simulink model "AOE_OBAS"  (R2024b)
settings: Solver=ode4  StartTime=0  StopTime=200  FixedStep=0.01  MaxStep=0.01  RelTol=1e-3
values from neighbouring files (symbols this model uses):
  AOE = Constants_3Body_v2(inputs)    [wecSimInputFile.m]
undefined symbols (not defined in the file or in its folder): body, constraint, DiscIntNeverNeededParam, pto
libraries: WECSim_Lib_Body_Elements x6, simulink x3, WECSim_Lib_Constraints x3, WECSim_Lib_PTOs x3, WECSim_Lib_Frames x1
(part 1 of 2)
settings Model: Creator=wcwi  LastModifiedBy=Luke
settings SolverCC: ZeroCrossControl=DisableAll  AlgebraicLoopSolver=TrustRegion  PositivePriorityOrder=on  AutoInsertRateTranBlk=on  InsertRTBMode=Never (minimum delay)
settings DataIOCC: SaveFormat=Array  ReturnWorkspaceOutputs=off
settings OptimizationCC: LifeSpan=inf  SimCompilerOptimization=on  AccelVerboseBuild=on
settings DebuggingCC: UnconnectedInputMsg=warning  UnconnectedOutputMsg=warning  UnconnectedLineMsg=warning  SFUnexpectedBacktrackingDiag=warning  SFNoUnconditionalDefaultTransitionDiag=warning  SFExecutionAtInitializationDiag=none  ArithmeticOperatorsInVariantConditions=warning
settings HardwareCC: ProdBitPerSizeT=32  ProdBitPerPtrDiffT=32  ProdWordSize=32  ProdHWDeviceType=Specified
settings ModelReferenceCC: UpdateModelReferenceTargets=Force  PropagateSignalLabelsOutOfModel=off
settings SFSimCC: SimUseLocalCustomCode=off  CustomCodeUndefinedFunction=UseInterfaceOnly
settings RTWCC: RTWUseLocalCustomCode=off  GPUComputeCapability=3.5
settings CodeAppCC: StateflowObjectComments=on
settings GRTTargetCC: TargetLangStandard=C89/C90 (ANSI)
settings ConfigComp: CovMetricSettings=dw  CovSaveCumulativeToWorkspaceVar=on  CovSaveSingleToWorkspaceVar=on  CovExternalEMLEnable=off

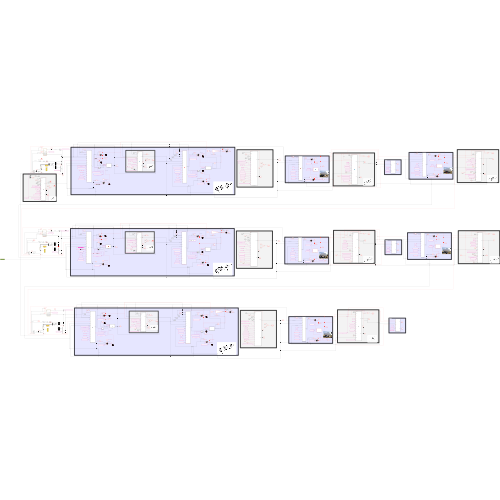
[thumbnail: Simulink's stored preview of the top-level diagram]
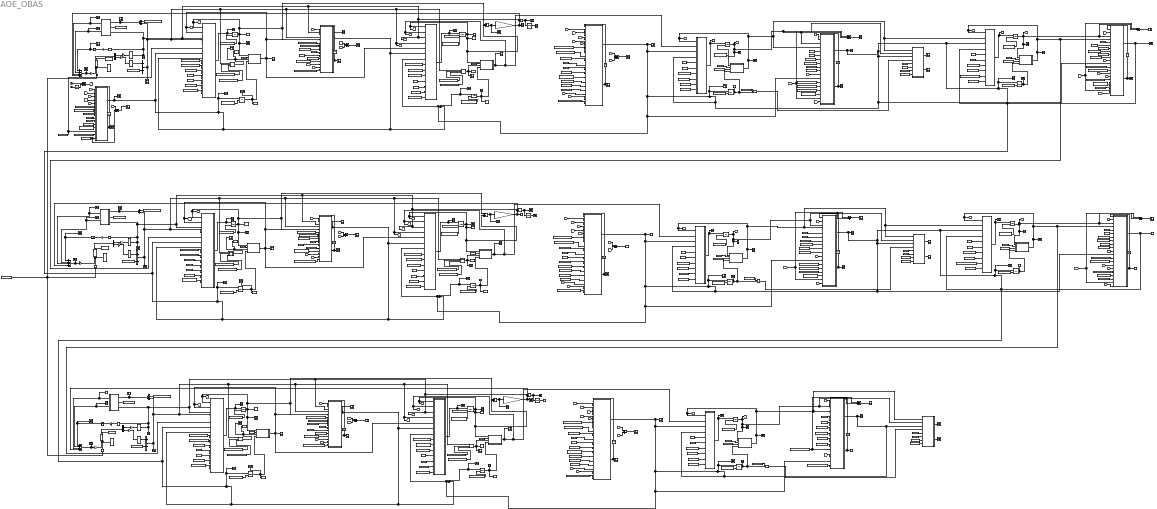
== system AOE_OBAS ==
  note: Outlet Piston Chamber 1 Valve
  note: Outlet Tank Valve
  note: Inlet Piston valve
  note: Outlet Piston Valve
  note: Outlet Piston Chamber 1 Valve
  note: Outlet Tank Valve
  note: Outlet Piston Valve
  note: Outlet Piston Chamber 1 Valve
  note: Outlet Tank Valve
  note: Outlet Piston Valve
  note: Useful Power
  note: Useful Power
  note: Useful Power
  note: Outlet Tank Valve
  note: Outlet Tank Valve
  " mdot Pipe U1U2" : Scope
  " mdot Pipe U2U3" : Scope
  " mdot Tank Unit1" : Scope
  " mdot Tank Unit2" : Scope
  " mdot Tank Unit3" : Scope
  " mdot max Pipe U1U2" : Scope
  " mdot max Pipe U2U3" : Scope
  " mdot max Tank Unit1" : Scope
  " mdot max Tank Unit2" : Scope
  " mdot max Tank Unit3" : Scope
  Add{1,13..15} (4 alike) : Sum  Inputs=+-
  Add{2..7,9..11,16..18} (12 alike) : Sum  Inputs=-+
  Add12 : Sum  Inputs=++++  RndMeth=Simplest
  Add19 : Sum  Inputs=++++  RndMeth=Simplest
  Add8 : Sum  Inputs=++++  RndMeth=Simplest
  Air Mass Chamber1 Unit1 : Scope
  Air Mass Chamber1 Unit2 : Scope
  Air Mass Chamber1 Unit3 : Scope
  Air Mass Chamber2 Unit1 : Scope
  Air Mass Chamber2 Unit2 : Scope
  Air Mass Chamber2 Unit3 : Scope
  Air Mass Pipe U1U2 : Scope
  Air Mass Pipe U2U3 : Scope
  Air Mass change rate Chamber1 Unit1 : Scope
  Air Mass change rate Chamber1 Unit2 : Scope
  Air Mass change rate Chamber1 Unit3 : Scope
  Air Mass change rate Chamber2 Unit1 : Scope
  Air Mass change rate Chamber2 Unit2 : Scope
  Air Mass change rate Chamber2 Unit3 : Scope
  Assertion : Assertion  AssertionFailFcn=Ch1C1 mass is zero
  Assertion1 : Assertion  AssertionFailFcn=Ch1C1 pressure is zero
  Assertion10 : Assertion  AssertionFailFcn=Ch1C1 volume is zero
  Assertion11 : Assertion  AssertionFailFcn=Ch2C1 volume is zero
  Assertion12 : Assertion  AssertionFailFcn=Ch1C1 mass is zero
  Assertion13 : Assertion  AssertionFailFcn=Ch1C1 pressure is zero
  Assertion14 : Assertion  AssertionFailFcn=Ch2C1 pressure is zero  StopWhenAssertionFail=off
  Assertion15 : Assertion  AssertionFailFcn=Ch2C1 mass is zero
  Assertion16 : Assertion  AssertionFailFcn=Ch1C1 volume is zero
  Assertion17 : Assertion  AssertionFailFcn=Ch2C1 volume is zero
  Assertion2 : Assertion  AssertionFailFcn=Ch2C1 pressure is zero  StopWhenAssertionFail=off
  Assertion3 : Assertion  AssertionFailFcn=Ch2C1 mass is zero
  Assertion4 : Assertion  AssertionFailFcn=Ch1C1 volume is zero
  Assertion5 : Assertion  AssertionFailFcn=Ch2C1 volume is zero
  Assertion6 : Assertion  AssertionFailFcn=Ch1C1 mass is zero
  Assertion7 : Assertion  AssertionFailFcn=Ch1C1 pressure is zero
  Assertion8 : Assertion  AssertionFailFcn=Ch2C1 pressure is zero  StopWhenAssertionFail=off
  Assertion9 : Assertion  AssertionFailFcn=Ch2C1 mass is zero
  Atmospheric pressure{1..4} (4 alike) : Constant  Value=AOE.AtmPressure
  Bus Selector : BusSelector  OutputSignals=velocity,position
  Bus Selector1 : BusSelector  OutputSignals=velocity,position
  Bus Selector2 : BusSelector  OutputSignals=velocity,position
  Chamber pressure potential Unit1 : Scope
  Chamber pressure potential Unit2 : Scope
  Chamber pressure potential Unit3 : Scope
  Clock : Clock
  Clock1 : Clock
  Constant{1,14,24,37,56} (5 alike) : Constant  Value=AOE.Unit1.Cylinder.HeatConvection
  Constant{2,10,71,85,208} (5 alike) : Constant  Value=AOE.Unit2.Cylinder.HeatConvection
  Constant{76,90,94,97,100,118,200} (7 alike) : Constant  Value=AOE.Unit2.Cylinder.CrossSectionalArea
  Constant{8,26,38,42,52,57,64,73,86,91,101,106,119,133,146,151,161,166,174,179,186,209,214} (23 alike) : Constant  Value=AOE.WaterTemperature
  Constant102 : Constant  Value=AOE.Unit2.Tank.HeatConvection
  Constant103 : Constant  Value=AOE.Unit2.Tank.SurfaceArea
  Constant{96,99,104,110} (4 alike) : Constant  Value=AOE.Unit2.Tank.Volume
  Constant105 : Constant  Value=AOE.Unit1.Pipe.CrossSectionalArea
  Constant107 : Constant  Value=AOE.Unit2.Tank.HeatConvection
  Constant108 : Constant  Value=AOE.Unit2.Tank.SurfaceArea
  Constant{6,23,28,31,40,47,62,70,75,79,89,95,109,130,135,139,149,155,169,181,198,203,213} (23 alike) : Constant  Value=AOE.gma
  Constant11 : Constant  Value=AOE.Unit2.Chamber2.InitialPistonPosition
  Constant111 : Constant  Value=AOE.Unit1.Pipe.HeatConvection
  Constant112 : Constant  Value=AOE.Unit2.Pipe.InitialAirMass
  Constant113 : Constant  Value=AOE.Unit2.Pipe.CrossSectionalArea
  Constant{3..5,22,27,30,35,39,43,61,69,74,77..78,83,87..88,92,98,114,129,134,137..138,143,147..148,152,158,165,172,175,185,197,202,207,211} (37 alike) : Constant  Value=AOE.Rs
  Constant115 : Constant  Value=AOE.Cp
  Constant116 : Constant  Value=AOE.Unit2.OutletCylinderOrifice.CrossSectionalArea
  Constant117 : Constant  Value=AOE.Unit2.Chamber1Chamber2Orifice.CrossSectionalArea
  Constant12 : Constant  Value=AOE.Unit2.Cylinder.Diameter
  Constant120 : Constant  Value=AOE.Unit2.Chamber1.InitialAirMass
  Constant{121..122,131,145,195} (5 alike) : Constant  Value=AOE.Unit3.Cylinder.HeatConvection
  Constant123 : Constant  Value=AOE.Unit3.Chamber2.InitialPistonPosition
  Constant124 : Constant  Value=AOE.Unit3.Cylinder.Diameter
  Constant125 : Constant  Value=AOE.Unit3.Chamber2.InitialAirMass
  Constant126 : Constant  Value=AOE.Unit3.Chamber1.InitialPressure
  Constant127 : Constant  Value=AOE.Unit3.Chamber2.InitialPressure
  Constant128 : Constant  Value=AOE.Unit3.OutletTankOrifice.CrossSectionalArea
  Constant13 : Constant  Value=AOE.Unit2.Chamber2.InitialAirMass
  Constant132 : Constant  Value=AOE.Unit3.Tank.InitialAirMass
  Constant{136,150,154,157,160,178,194} (7 alike) : Constant  Value=AOE.Unit3.Cylinder.CrossSectionalArea
  Constant140 : Constant  Value=AOE.Unit3.Tank.HeatConvection
  Constant141 : Constant  Value=AOE.Unit3.Tank.InitialPressure
  Constant142 : Constant  Value=AOE.Unit3.Tank.SurfaceArea
  Constant{36,48,50,55,60,84,144} (7 alike) : Constant  Value=AOE.Unit1.Tank.Volume
  Constant15 : Constant  Value=AOE.Unit2.Chamber1.InitialPressure
  Constant153 : Constant  Value=AOE.Unit3.Chamber2.InitialPistonPosition
  Constant{156,159,164,170} (4 alike) : Constant  Value=AOE.Unit3.Tank.Volume
  Constant16 : Constant  Value=AOE.Unit1.Chamber2.InitialPistonPosition
  Constant162 : Constant  Value=AOE.Unit3.Tank.HeatConvection
  Constant163 : Constant  Value=AOE.Unit3.Tank.SurfaceArea
  Constant167 : Constant  Value=AOE.Unit3.Tank.HeatConvection
  Constant168 : Constant  Value=AOE.Unit3.Tank.SurfaceArea
  Constant17 : Constant  Value=AOE.Unit1.Cylinder.Diameter
  Constant171 : Constant  Value=AOE.Cp
  Constant173 : Constant  Value=AOE.Cp
  Constant176 : Constant  Value=AOE.Unit3.OutletCylinderOrifice.CrossSectionalArea
  Constant177 : Constant  Value=AOE.Unit3.Chamber1Chamber2Orifice.CrossSectionalArea
  Constant18 : Constant  Value=AOE.Unit1.Chamber2.InitialAirMass
  Constant180 : Constant  Value=AOE.Unit3.Chamber1.InitialAirMass
  Constant182 : Constant  Value=AOE.Unit2.Pipe.HeatConvection
  Constant183 : Constant  Value=AOE.Unit2.Pipe.InitialPressure
  Constant184 : Constant  Value=AOE.Unit2.Pipe.SurfaceArea
  Constant{187..188,193,199} (4 alike) : Constant  Value=AOE.Unit2.Pipe.Volume
  Constant189 : Constant  Value=AOE.Unit2.Pipe.HeatConvection
  Constant19 : Constant  Value=AOE.Unit1.Chamber1.InitialPressure
  Constant190 : Constant  Value=AOE.Unit2.Pipe.SurfaceArea
  Constant191 : Constant  Value=AOE.Unit2.Pipe.HeatConvection
  Constant196 : Constant  Value=AOE.Unit2.OutletPipeOrifice.CrossSectionalArea
  Constant20 : Constant  Value=AOE.Unit1.Chamber2.InitialPressure
  Constant201 : Constant  Value=AOE.Unit1.Pipe.InitialAirMass
  Constant204 : Constant  Value=AOE.Unit1.Pipe.HeatConvection
  Constant205 : Constant  Value=AOE.Unit1.Pipe.InitialPressure
  Constant206 : Constant  Value=AOE.Unit1.Pipe.SurfaceArea
  Constant21 : Constant  Value=AOE.Unit1.OutletTankOrifice.CrossSectionalArea
  Constant210 : Constant  Value=AOE.Unit1.OutletPipeOrifice.CrossSectionalArea
  Constant{212,217..218,220} (4 alike) : Constant  Value=AOE.Unit1.Pipe.Volume
  Constant215 : Constant  Value=AOE.Unit1.Pipe.HeatConvection
  Constant216 : Constant  Value=AOE.Unit1.Pipe.SurfaceArea
  Constant25 : Constant  Value=AOE.Unit1.Tank.InitialAirMass
  Constant{7,29,41,46,49,51,63} (7 alike) : Constant  Value=AOE.Unit1.Cylinder.CrossSectionalArea
  Constant32 : Constant  Value=AOE.Unit1.Tank.HeatConvection
  Constant33 : Constant  Value=AOE.Unit1.Tank.InitialPressure
  Constant34 : Constant  Value=AOE.Unit1.Tank.SurfaceArea
  Constant44 : Constant  Value=AOE.Unit1.Chamber2.InitialPistonPosition
  Constant45 : Constant  Value=AOE.Unit2.Chamber2.InitialPressure
  Constant53 : Constant  Value=AOE.Unit1.Tank.HeatConvection
  Constant54 : Constant  Value=AOE.Unit1.Tank.SurfaceArea
  Constant58 : Constant  Value=AOE.Unit1.Tank.HeatConvection
  Constant59 : Constant  Value=AOE.Unit1.Tank.SurfaceArea
  Constant65 : Constant  Value=AOE.Unit1.InletCylinderOrifice.CrossSectionalArea
  Constant66 : Constant  Value=AOE.Unit1.OutletCylinderOrifice.CrossSectionalArea
  Constant67 : Constant  Value=AOE.Unit1.Chamber1Chamber2Orifice.CrossSectionalArea
  Constant68 : Constant  Value=AOE.Unit2.OutletTankOrifice.CrossSectionalArea
  Constant72 : Constant  Value=AOE.Unit2.Tank.InitialAirMass
  Constant80 : Constant  Value=AOE.Unit2.Tank.HeatConvection
  Constant81 : Constant  Value=AOE.Unit2.Tank.InitialPressure
  Constant82 : Constant  Value=AOE.Unit2.Tank.SurfaceArea
  Constant9 : Constant  Value=AOE.Unit1.Chamber1.InitialAirMass
  Constant93 : Constant  Value=AOE.Unit2.Chamber2.InitialPistonPosition
  Coulomb & Viscous Friction Unit1 : simulink/Discontinuities/Coulomb & Viscous Friction  offset=0  gain=AOE.Unit1.Cylinder.CoulombFrictionGain
  Coulomb & Viscous Friction Unit2 : simulink/Discontinuities/Coulomb & Viscous Friction  offset=0  gain=AOE.Unit1.Cylinder.CoulombFrictionGain
  Coulomb & Viscous Friction Unit3 : simulink/Discontinuities/Coulomb & Viscous Friction  offset=0  gain=AOE.Unit1.Cylinder.CoulombFrictionGain
  Cyl D{,1..3} (4 alike) : Constant  Value=AOE.Unit1.Cylinder.Diameter
  Cyl D{6,8..9,11} (4 alike) : Constant  Value=AOE.Unit3.Cylinder.Diameter
  Cyl D{4..5,7,13} (4 alike) : Constant  Value=AOE.Unit2.Cylinder.Diameter
  Determining Useful Energy : MATLAB Function
      settings: MinAlgLoopOccurrences=on
  Determining Useful Energy1 : MATLAB Function
      settings: MinAlgLoopOccurrences=on
  Determining Useful Energy2 : MATLAB Function
      settings: MinAlgLoopOccurrences=on
  Discrete-Time Integrator{,1,3,5,8,12..15,18,21} (11 alike) : DiscreteIntegrator  InitialConditionSource=external  InitialCondition=101.3  SampleTime=-1  LimitOutput=on  LowerSaturationLimit=0  ICPrevOutput=DiscIntNeverNeededParam  ICPrevScaledInput=DiscIntNeverNeededParam
  Discrete-Time Integrator{4,6,10,16,20} (5 alike) : DiscreteIntegrator  InitialConditionSource=external  InitialCondition=1.2754*(10)*.25*pi*0.5^2  SampleTime=-1  LimitOutput=on  LowerSaturationLimit=0  ICPrevOutput=DiscIntNeverNeededParam  ICPrevScaledInput=DiscIntNeverNeededParam
  Discrete-Time Integrator{2,7,9,11,17,19} (6 alike) : DiscreteIntegrator  InitialConditionSource=external  InitialCondition=1.2754*(2+.05)*.25*pi*2.14^2  SampleTime=-1  LimitOutput=on  LowerSaturationLimit=0  ICPrevOutput=DiscIntNeverNeededParam  ICPrevScaledInput=DiscIntNeverNeededParam
  Endstop Forces Unit1 : Subsystem
  Endstop Forces Unit2 : Subsystem
  Endstop Forces Unit3 : Subsystem
  Energy : DiscreteIntegrator  SampleTime=-1  LimitOutput=on  ICPrevOutput=DiscIntNeverNeededParam  ICPrevScaledInput=DiscIntNeverNeededParam
  Energy Unit1 : Scope
  Energy Unit2 : Scope
  Energy Unit3 : Scope
  Energy1 : DiscreteIntegrator  SampleTime=-1  LimitOutput=on  ICPrevOutput=DiscIntNeverNeededParam  ICPrevScaledInput=DiscIntNeverNeededParam
  Energy2 : DiscreteIntegrator  SampleTime=-1  LimitOutput=on  ICPrevOutput=DiscIntNeverNeededParam  ICPrevScaledInput=DiscIntNeverNeededParam
  Exergy Unit1 : Scope
  Exergy Unit2 : Scope
  Exergy Unit3 : Scope
  Float : WECSim_Lib_Body_Elements/Rigid Body  body=body(1)
  Float1 : WECSim_Lib_Body_Elements/Rigid Body  body=body(3)
  Float2 : WECSim_Lib_Body_Elements/Rigid Body  body=body(5)
  Floating (6DOF) : WECSim_Lib_Constraints/Floating (6DOF)  constraint=constraint(1)
      settings: AttributesFormatString=%<constraint>
  Floating (6DOF)1 : WECSim_Lib_Constraints/Floating (6DOF)  constraint=constraint(2)
      settings: AttributesFormatString=%<constraint>
  Floating (6DOF)2 : WECSim_Lib_Constraints/Floating (6DOF)  constraint=constraint(3)
      settings: AttributesFormatString=%<constraint>
  Gain{,2,4,6..14} (12 alike) : Gain  Gain=-1
  Gain1 : Gain  Gain=AOE.Unit1.Cylinder.CrossSectionalArea
  Gain3 : Gain  Gain=AOE.Unit2.Cylinder.CrossSectionalArea
  Gain5 : Gain  Gain=AOE.Unit3.Cylinder.CrossSectionalArea
  Global Reference Frame : WECSim_Lib_Frames/Global Reference Frame  waves=waves  simu=simu
      settings: SourceProductName=WEC-Sim
  Mech_Energy Unit1 : Scope
  Mech_Energy Unit2 : Scope
  Mech_Energy Unit3 : Scope
  Mech_FTO Unit1 : Scope
  Mech_FTO Unit2 : Scope
  Mech_FTO Unit3 : Scope
  Mech_PTO Unit1 : Scope
  Mech_PTO Unit2 : Scope
  Mech_PTO Unit3 : Scope
  PTO Friction Unit1 : Scope
  PTO Friction Unit2 : Scope
  PTO Friction Unit3 : Scope
  Pdot Chamber1 Unit1 : Scope
  Pdot Chamber1 Unit2 : Scope
  Pdot Chamber1 Unit3 : Scope
  Pdot Chamber2 Unit1 : Scope
  Pdot Chamber2 Unit2 : Scope
  Pdot Chamber2 Unit3 : Scope
  Pdot Pipe U1U2 : Scope
  Pdot Pipe U2U3 : Scope
  Pdot Tank Unit1 : Scope
  Pdot Tank Unit2 : Scope
  Pdot Tank Unit3 : Scope
  Pipe Air Mass change rate U1U2 : Scope
  Pipe Air Mass change rate U2U3 : Scope
  Pipe Unit1 to Unit1 : MATLAB Function
      settings: MinAlgLoopOccurrences=on
  Pipe Unit1 to Unit2 : MATLAB Function
      settings: MinAlgLoopOccurrences=on
  Pressure Chamber1 Box Unit1 : MATLAB Function
      settings: MinAlgLoopOccurrences=on
  Pressure Chamber1 Box Unit2 : MATLAB Function
      settings: MinAlgLoopOccurrences=on
  Pressure Chamber1 Box Unit3 : MATLAB Function
      settings: MinAlgLoopOccurrences=on
  Pressure Chamber1 Unit1 : Scope
  Pressure Chamber1 Unit2 : Scope
  Pressure Chamber1 Unit3 : Scope
  Pressure Chamber2 Box Unit1 : MATLAB Function
  Pressure Chamber2 Box Unit2 : MATLAB Function
  Pressure Chamber2 Box Unit3 : MATLAB Function
  Pressure Chamber2 Unit1 : Scope
  Pressure Chamber2 Unit2 : Scope
  Pressure Chamber2 Unit3 : Scope
  Pressure Difference Chamb. 1 Unit1 : Scope
  Pressure Difference Chamb. 1 Unit2 : Scope
  Pressure Difference Chamb. 1 Unit3 : Scope
  Pressure Difference Cyl. Unit1 : Scope
  Pressure Difference Cyl. Unit2 : Scope
  Pressure Difference Cyl. Unit3 : Scope
  Pressure Difference Inlet Unit1 : Scope
  Pressure Difference Pipe U2U3 : Scope
  Pressure Difference Pipe Unit1 : Scope
  Pressure Difference Tank Unit1 : Scope
  Pressure Difference Tank Unit2 : Scope
  Pressure Difference Tank Unit3 : Scope
  Pressure Pipe U1U2 : Scope
  Pressure Pipe U2U3 : Scope
  Pressure Tank Box Unit1 : MATLAB Function
      settings: MinAlgLoopOccurrences=on
  Pressure Tank Box Unit2 : MATLAB Function
      settings: MinAlgLoopOccurrences=on
  Pressure Tank Box Unit3 : MATLAB Function
      settings: MinAlgLoopOccurrences=on
  Pressure Tank Unit1 : Scope
  Pressure Tank Unit2 : Scope
  Pressure Tank Unit3 : Scope
  Product1 : Product  Inputs=/*
  Product2 : Product
  Product3 : Product  Inputs=/*
  Product4 : Product  Inputs=/*
  Product5 : Product
  Product8 : Product
  Revised Valve Model : MATLAB Function
      settings: MinAlgLoopOccurrences=on
  Revised Valve Model Chamber1Chamber2 Unit1 : MATLAB Function
      settings: MinAlgLoopOccurrences=on
  Revised Valve Model Chamber1Chamber2 Unit2 : MATLAB Function
      settings: MinAlgLoopOccurrences=on
  Revised Valve Model Chamber1Chamber2 Unit3 : MATLAB Function
      settings: MinAlgLoopOccurrences=on
  Revised Valve Model Inlet Unit1 : MATLAB Function
      settings: MinAlgLoopOccurrences=on
  Revised Valve Model Piston Outlet Unit2 : MATLAB Function
      settings: MinAlgLoopOccurrences=on
  Revised Valve Model Piston Outlet Unit3 : MATLAB Function
      settings: MinAlgLoopOccurrences=on
  Revised Valve Pipe Outlet Unit1 : MATLAB Function
      settings: MinAlgLoopOccurrences=on
  Revised Valve Pipe Outlet Unit2 : MATLAB Function
      settings: MinAlgLoopOccurrences=on
  Revised Valve Tank Outlet Unit1 : MATLAB Function
      settings: MinAlgLoopOccurrences=on
  Revised Valve Tank Outlet Unit2 : MATLAB Function
      settings: MinAlgLoopOccurrences=on
  Revised Valve Tank Outlet2 : MATLAB Function
      settings: MinAlgLoopOccurrences=on
  Saturation : Saturate  UpperLimit=AOE.Unit1.Cylinder.CoulombFrictionLimit  LowerLimit=-AOE.Unit1.Cylinder.CoulombFrictionLimit
  Saturation1 : Saturate  UpperLimit=AOE.Unit1.Cylinder.CoulombFrictionLimit  LowerLimit=-AOE.Unit1.Cylinder.CoulombFrictionLimit
  Saturation2 : Saturate  UpperLimit=AOE.Unit1.Cylinder.CoulombFrictionLimit  LowerLimit=-AOE.Unit1.Cylinder.CoulombFrictionLimit
  Selector{,1..5} (6 alike) : Selector  InputPortWidth=6  IndexOptions=Index vector (dialog)  Indices=3  OutputSizes=1
  Spar : WECSim_Lib_Body_Elements/Rigid Body  body=body(2)
  Spar1 : WECSim_Lib_Body_Elements/Rigid Body  body=body(4)
  Spar2 : WECSim_Lib_Body_Elements/Rigid Body  body=body(6)
  Sum : Sum  Inputs=+-
  Sum{1..2,5,7,11..12} (6 alike) : Sum  Inputs=-+
  Sum10 : Sum  Inputs=+-
  Sum{3,8,13,15..16} (5 alike) : Sum  Inputs=+|-
  Sum14 : Sum
  Sum4 : Sum  Inputs=+-
  Sum6 : Sum
  Sum9 : Sum
  Tank Air Mass Unit1 : Scope
  Tank Air Mass Unit2 : Scope
  Tank Air Mass Unit3 : Scope
  Tank Air Mass change rate Unit1 : Scope
  Tank Air Mass change rate Unit2 : Scope
  Tank Air Mass change rate Unit3 : Scope
  Temp Chamber1 Unit1 : Scope
  Temp Chamber1 Unit2 : Scope
  Temp Chamber1 Unit3 : Scope
  Temp Chamber2 Unit1 : Scope
  Temp Chamber2 Unit2 : Scope
  Temp Chamber2 Unit3 : Scope
  Temp Pipe U1U2 : Scope
  Temp Pipe U2U3 : Scope
  Temp Tank Unit1 : Scope
  Temp Tank Unit2 : Scope
  Temp Tank Unit3 : Scope
  Temperature Chamber1 Box Unit1 : MATLAB Function  TreatAsAtomicUnit=on
      settings: MinAlgLoopOccurrences=on
  Temperature Chamber1 Box Unit2 : MATLAB Function  TreatAsAtomicUnit=on
      settings: MinAlgLoopOccurrences=on
  Temperature Chamber1 Box Unit3 : MATLAB Function  TreatAsAtomicUnit=on
      settings: MinAlgLoopOccurrences=on
  Temperature Chamber2 Box Unit1 : MATLAB Function
      settings: MinAlgLoopOccurrences=on
  Temperature Chamber2 Box Unit2 : MATLAB Function
      settings: MinAlgLoopOccurrences=on
  Temperature Chamber2 Box Unit3 : MATLAB Function
      settings: MinAlgLoopOccurrences=on
  Temperature Pipe Unit1 to Unit1 : MATLAB Function
  Temperature Pipe Unit1 to Unit2 : MATLAB Function
  Temperature Tank Box Unit1 : MATLAB Function
  Temperature Tank Box Unit2 : MATLAB Function
  Temperature Tank Box Unit3 : MATLAB Function
  Total Reaction Force : Scope
  Total Reaction Force1 : Scope
  Total Reaction Force2 : Scope
  Translational PTO Actuation Force : WECSim_Lib_PTOs/Translational PTO Actuation Force  pto=pto(1)
      settings: AttributesFormatString=%<pto>
  Translational PTO Actuation Force1 : WECSim_Lib_PTOs/Translational PTO Actuation Force  pto=pto(2)
      settings: AttributesFormatString=%<pto>
  Translational PTO Actuation Force2 : WECSim_Lib_PTOs/Translational PTO Actuation Force  pto=pto(3)
      settings: AttributesFormatString=%<pto>
  Unit Delay{,1..12} (13 alike) : UnitDelay  SampleTime=-1  HasFrameUpgradeWarning=on
  Vol Chamber1 Unit1 : Scope
  Vol Chamber1 Unit2 : Scope
  Vol Chamber1 Unit3 : Scope
  Vol Chamber2 Unit1 : Scope
  Vol Chamber2 Unit2 : Scope
  Vol Chamber2 Unit3 : Scope
  Volume Chamber1 Box Unit1 : MATLAB Function  TreatAsAtomicUnit=on
      settings: MinAlgLoopOccurrences=on
  Volume Chamber1 Box Unit2 : MATLAB Function  TreatAsAtomicUnit=on
      settings: MinAlgLoopOccurrences=on
  Volume Chamber1 Box Unit3 : MATLAB Function  TreatAsAtomicUnit=on
      settings: MinAlgLoopOccurrences=on
  Volume Chamber2 Box Unit1 : MATLAB Function  TreatAsAtomicUnit=on
      settings: MinAlgLoopOccurrences=on
  Volume Chamber2 Box Unit2 : MATLAB Function  TreatAsAtomicUnit=on
      settings: MinAlgLoopOccurrences=on
  Volume Chamber2 Box Unit3 : MATLAB Function  TreatAsAtomicUnit=on
      settings: MinAlgLoopOccurrences=on
  cylinder equilibrium offset position{1,3..5} (4 alike) : Constant  Value=AOE.Unit1.Chamber1.InitialPistonPosition
  cylinder equilibrium offset position{7,9..10,20} (4 alike) : Constant  Value=AOE.Unit2.Chamber1.InitialPistonPosition
  cylinder equilibrium offset position{11,13,15..16} (4 alike) : Constant  Value=AOE.Unit3.Chamber1.InitialPistonPosition
  cylinder equilibrium offset position12 : Constant  Value=AOE.Unit2.Chamber2.InitialPistonPosition
  cylinder equilibrium offset position14 : Constant  Value=AOE.Unit3.Chamber2.InitialPistonPosition
  cylinder equilibrium offset position18 : Constant  Value=AOE.Unit3.Chamber2.InitialPistonPosition
  cylinder equilibrium offset position2 : Constant  Value=AOE.Unit1.Chamber2.InitialPistonPosition
  cylinder equilibrium offset position6 : Constant  Value=AOE.Unit1.Chamber2.InitialPistonPosition
  cylinder equilibrium offset position8 : Constant  Value=AOE.Unit2.Chamber2.InitialPistonPosition
  cylinder total Length : Constant  Value=AOE.Unit1.Cylinder.Length
  cylinder total Length1 : Constant  Value=AOE.Unit2.Cylinder.Length
  cylinder total Length2 : Constant  Value=AOE.Unit3.Cylinder.Length
  cylinder total Length3 : Constant  Value=AOE.Unit1.Cylinder.InitialOffset
  cylinder total Length4 : Constant  Value=AOE.Unit1.Cylinder.InitialOffset
  cylinder total Length5 : Constant  Value=AOE.Unit1.Cylinder.InitialOffset
  joint F stop high Unit1 : Scope
  joint F stop high Unit2 : Scope
  joint F stop high Unit3 : Scope
  joint F stop low Unit1 : Scope
  joint F stop low Unit2 : Scope
  joint F stop low Unit3 : Scope
  joint position1 : Scope
  joint position2 : Scope
  joint position3 : Scope
  mdot Chamber1Chamber2 Unit1 : Scope
  mdot Chamber1Chamber2 Unit2 : Scope
  mdot Chamber1Chamber2 Unit3 : Scope
  mdot Cylinder Unit1 : Scope
  mdot Cylinder Unit2 : Scope
  mdot Cylinder Unit3 : Scope
  mdot Inlet Unit1 : Scope
  mdot Max Chamber1Chamber2 Unit1 : Scope
  mdot Max Chamber1Chamber2 Unit2 : Scope
  mdot Max Chamber1Chamber2 Unit3 : Scope
  mdot Max Cylinder Unit1 : Scope
  mdot Max Cylinder Unit2 : Scope
  mdot Max Cylinder Unit3 : Scope
  mdot max Inlet Unit1 : Scope
  override3 : Constant  Value=AOE.Unit3.OutletTankCheckValve.CrackPressure
  piston position Unit1 : Scope
  piston position Unit2 : Scope
  piston position Unit3 : Scope
  piston velocity Unit2 : Scope
  piston velocity Unit3 : Scope
  piston velocity Unit4 : Scope
  tempAmb{1..4} (4 alike) : Constant  Value=AOE.AtmTemperature
  wires:
  Coulomb & Viscous Friction Unit1/1 -> Gain/1
  Saturation/1 -> PTO Friction Unit1/1, Add8/1  "Motion Friction"
  Endstop Forces Unit1/2(F_stop_lo) -> joint F stop low Unit1/1, Add8/2  "Fstop_low"
  cylinder total Length/1 -> Endstop Forces Unit1/2(Total length)
  Sum6/1 -> Endstop Forces Unit1/1(x(t)), joint position1/1  "Piston Position"
  Endstop Forces Unit1/1(F_stop_hi) -> joint F stop high Unit1/1, Add8/3  "Fstop_high"
  Gain/1 -> Saturation/1
  Constant44/1 -> Sum6/1
  Add13/1 -> piston position Unit1/1, Volume Chamber1 Box Unit1/1(x), Revised Valve Model Chamber1Chamber2 Unit1/4(x), Pressure Chamber2 Box Unit1/4(x), [x], Volume Chamber2 Box Unit1/1(x), Pressure Chamber1 Box Unit1/4(x), Sum6/2  "x"
  Pressure Chamber1 Box Unit1/1(Pdot) -> Pdot Chamber1 Unit1/1, Discrete-Time Integrator/1  "pdot(t)"
  Sum/1 -> Discrete-Time Integrator11/1, Air Mass change rate Chamber1 Unit1/1  "mdot1-mdot2"
  Discrete-Time Integrator11/1 -> Air Mass Chamber1 Unit1/1, Temperature Chamber1 Box Unit1/4(m), Assertion/1  "chamber1 air mass"
  Discrete-Time Integrator/1 -> Pressure Chamber1 Box Unit1/1(P), [PC1], Revised Valve Model Chamber1Chamber2 Unit1/5(PC1), Sum1/1, Assertion1/1, Pressure Chamber1 Unit1/1, Temperature Chamber1 Box Unit1/1(P)  "Chamber1 Pressure"
  cylinder equilibrium offset position4/1 -> Pressure Chamber1 Box Unit1/8(L)
  Cyl D/1 -> Pressure Chamber1 Box Unit1/10(D)
  Constant9/1 -> Discrete-Time Integrator11/2
  Constant5/1 -> Pressure Chamber1 Box Unit1/11(Rs)
  Constant6/1 -> Pressure Chamber1 Box Unit1/12(gma)
  Constant7/1 -> Pressure Chamber1 Box Unit1/9(A)
  Constant8/1 -> Pressure Chamber1 Box Unit1/13(Tw)
  Constant37/1 -> Pressure Chamber1 Box Unit1/14(h)
  Constant19/1 -> Discrete-Time Integrator/2
  Constant3/1 -> Temperature Chamber1 Box Unit1/2(Rs)
  Revised Valve Model Chamber1Chamber2 Unit1/1(MassFlow) -> mdot Chamber1Chamber2 Unit1/1, Sum2/2, Pressure Chamber1 Box Unit1/7(mdot3), Sum/2, Pressure Chamber2 Box Unit1/6(mdot1)  "mdot(t)"
  Pressure Chamber2 Box Unit1/1(Pdot) -> Pdot Chamber2 Unit1/1, Discrete-Time Integrator12/1  "pdot(t)"
  Volume Chamber2 Box Unit1/1(V) -> Vol Chamber2 Unit1/1, Assertion5/1, Temperature Chamber2 Box Unit1/3(V)  "Chamber2 volume"
  Sum2/1 -> Discrete-Time Integrator2/1, Air Mass change rate Chamber2 Unit1/1
  Discrete-Time Integrator2/1 -> Temperature Chamber2 Box Unit1/4(m), Air Mass Chamber2 Unit1/1, Assertion3/1  "Chamber2 air mass"
  Constant18/1 -> Discrete-Time Integrator2/2
  Temperature Chamber2 Box Unit1/1(T) -> Temp Chamber2 Unit1/1, Pressure Chamber2 Box Unit1/2(T), [TC2], Pressure Tank Box Unit1/2(Tin)  "Chamber2 temperature"
  Constant16/1 -> Pressure Chamber2 Box Unit1/8(L)
  Constant17/1 -> Pressure Chamber2 Box Unit1/10(D)
  Constant20/1 -> Discrete-Time Integrator12/2
  Constant24/1 -> Pressure Chamber2 Box Unit1/14(h)
  Constant27/1 -> Pressure Chamber2 Box Unit1/11(Rs)
  Constant28/1 -> Pressure Chamber2 Box Unit1/12(gma)
  Constant29/1 -> Pressure Chamber2 Box Unit1/9(A)
  Constant26/1 -> Pressure Chamber2 Box Unit1/13(Tw)
  Constant4/1 -> Temperature Chamber2 Box Unit1/2(Rs)
  Temperature Chamber1 Box Unit1/1(T) -> Pressure Chamber2 Box Unit1/5(Tin1), Temp Chamber1 Unit1/1, Pressure Chamber1 Box Unit1/2(T), [TC1], Revised Valve Model Chamber1Chamber2 Unit1/6(TC1)  "chamber1 temp"
  Revised Valve Model/1(MassFlow) -> Revised Valve Tank Outlet Unit1/12(mDotIn), Pressure Chamber2 Box Unit1/7(mdot3), Sum2/1, Sum3/1, Pressure Tank Box Unit1/3(mdot1), mdot Cylinder Unit1/1  "Outlet cylinder"
  Gain1/1 -> Add8/4, Product2/2, Mech_FTO Unit1/1  "Pressure Potential Force"
  Sum1/1 -> Chamber pressure potential Unit1/1, Gain1/1
  Product2/1 -> Energy/1, Mech_PTO Unit1/1
  Energy/1 -> Mech_Energy Unit1/1
  Discrete-Time Integrator12/1 -> Pressure Chamber2 Box Unit1/1(P), [PC2], Pressure Chamber2 Unit1/1, Assertion2/1, Temperature Chamber2 Box Unit1/1(P), Sum1/2  "Chamber2 Pressure"
  Volume Chamber1 Box Unit1/1(V) -> Vol Chamber1 Unit1/1, Assertion4/1, Temperature Chamber1 Box Unit1/3(V)  "Chamber1 Volume"
  cylinder equilibrium offset position1/1 -> Volume Chamber1 Box Unit1/3(L)
  Constant46/1 -> Volume Chamber1 Box Unit1/2(A)
  cylinder equilibrium offset position2/1 -> Volume Chamber2 Box Unit1/3(L)
  Constant49/1 -> Volume Chamber2 Box Unit1/2(A)
  Pressure Tank Box Unit1/1(Pdot) -> Pdot Tank Unit1/1, Discrete-Time Integrator1/1
  Sum3/1 -> Tank Air Mass change rate Unit1/1, Discrete-Time Integrator10/1  "mdot1-mdot2"
  Discrete-Time Integrator10/1 -> Product1/2, Temperature Tank Box Unit1/4(m), Tank Air Mass Unit1/1  "Tank air mas"
  Constant25/1 -> Discrete-Time Integrator10/2
  Constant30/1 -> Pressure Tank Box Unit1/5(Rs)
  Constant31/1 -> Pressure Tank Box Unit1/6(gma)
  Constant32/1 -> Pressure Tank Box Unit1/7(h)
  Constant33/1 -> Discrete-Time Integrator1/2
  Constant34/1 -> Pressure Tank Box Unit1/8(a)
  Constant38/1 -> Pressure Tank Box Unit1/10(Tw)
  Constant50/1 -> Pressure Tank Box Unit1/9(V)
  Constant35/1 -> Temperature Tank Box Unit1/2(Rs)
  Constant48/1 -> Temperature Tank Box Unit1/3(V)
  Temperature Tank Box Unit1/1(T) -> Temp Tank Unit1/1, Revised Valve Tank Outlet Unit1/4(TT), Determining Useful Energy/1(T), Pipe Unit1 to Unit2/2(Tin), Pressure Tank Box Unit1/1(T), [TT]  "Unit1 Tank temp"
  Discrete-Time Integrator1/1 -> [PT], Temperature Tank Box Unit1/1(P), Pressure Tank Unit1/1, Add3/2, Revised Valve Tank Outlet Unit1/3(PT), Determining Useful Energy/2(P)  "Tank pressure"
  Constant14/1 -> Revised Valve Model/13(hC)
  Constant52/1 -> Revised Valve Model/12(Tw)
  Constant47/1 -> Revised Valve Model/11(gma)
  Constant43/1 -> Revised Valve Model/10(Rs)
  Cyl D1/1 -> Revised Valve Model/9(DC)
  Constant51/1 -> Revised Valve Model/8(AC)
  cylinder equilibrium offset position6/1 -> Revised Valve Model/7(LC)
  Clock1/1 -> Unit Delay1/1
  Unit Delay1/1 -> Add1/2
  Clock/1 -> Add1/1
  Add1/1 -> [TimeStep]
  [TimeStep] -> Revised Valve Model/2(TimeStep)
  Constant53/1 -> Revised Valve Model/14(hT)
  Constant54/1 -> Revised Valve Model/15(aT)
  Constant55/1 -> Revised Valve Model/16(VT)
  [PC2] -> Revised Valve Model/3(PC)
  [TC2] -> Revised Valve Model/4(TC)
  [xDot] -> Revised Valve Model/5(xdot)
  [x] -> Revised Valve Model/6(x)
  [TT] -> Revised Valve Model/18(TT)
  [PT] -> Add2/1
  [PC2] -> Add2/2
  Add2/1 -> Pressure Difference Cyl. Unit1/1
  [PT] -> Revised Valve Model/17(PT)
  [TimeStep] -> Revised Valve Tank Outlet Unit1/2(TimeStep)
  Constant57/1 -> Revised Valve Tank Outlet Unit1/7(Tw)
  Constant23/1 -> Revised Valve Tank Outlet Unit1/6(gma)
  Constant22/1 -> Revised Valve Tank Outlet Unit1/5(Rs)
  Constant58/1 -> Revised Valve Tank Outlet Unit1/8(hT)
  Constant59/1 -> Revised Valve Tank Outlet Unit1/10(aT)
  Constant60/1 -> Revised Valve Tank Outlet Unit1/9(VT)
  [TC2] -> Revised Valve Tank Outlet Unit1/11(TC)
  Revised Valve Tank Outlet Unit1/1(MassFlow) -> " mdot Tank Unit1"/1, Determining Useful Energy/3(mDot), Sum3/2, Pressure Tank Box Unit1/4(mdot2), Revised Valve Pipe Outlet Unit1/12(mDotIn), Sum16/1, Pipe Unit1 to Unit2/3(mdot1)  "Unit1 Outlet tank mdot"
  Constant21/1 -> Revised Valve Tank Outlet Unit1/13(A)
  Revised Valve Tank Outlet Unit1/2(mdotMax) -> Unit Delay/1, " mdot max Tank Unit1"/1
  Revised Valve Model Inlet Unit1/1(MassFlow) -> Sum/1, Pressure Chamber1 Box Unit1/6(mdot1), mdot Inlet Unit1/1  "Inlet Cylinder MassFlow to Cyl"
  Constant56/1 -> Revised Valve Model Inlet Unit1/13(hC)
  Constant64/1 -> Revised Valve Model Inlet Unit1/12(Tw)
  Constant62/1 -> Revised Valve Model Inlet Unit1/11(gma)
  Constant61/1 -> Revised Valve Model Inlet Unit1/10(Rs)
  Cyl D2/1 -> Revised Valve Model Inlet Unit1/9(DC)
  Constant63/1 -> Revised Valve Model Inlet Unit1/8(AC)
  cylinder equilibrium offset position5/1 -> Revised Valve Model Inlet Unit1/7(LC)
  [TimeStep] -> Revised Valve Model Inlet Unit1/2(TimeStep)
  [PC1] -> Revised Valve Model Inlet Unit1/3(PC1)
  [TC1] -> Revised Valve Model Inlet Unit1/4(TC1)
  [xDot] -> Revised Valve Model Inlet Unit1/5(xdot)
  [x] -> Revised Valve Model Inlet Unit1/6(x)
  Constant65/1 -> Revised Valve Model Inlet Unit1/15(A)
  tempAmb1/1 -> Revised Valve Model Inlet Unit1/14(Tamb), Pressure Chamber1 Box Unit1/5(Tin1)
  Atmospheric pressure1/1 -> Revised Valve Model Inlet Unit1/16(Pamb), Add9/2
  Revised Valve Model Inlet Unit1/2(mdotMax) -> Unit Delay4/1, mdot max Inlet Unit1/1
  Constant66/1 -> Revised Valve Model/19(A)
  cylinder equilibrium offset position3/1 -> Revised Valve Model Chamber1Chamber2 Unit1/7(LC)
  Cyl D3/1 -> Revised Valve Model Chamber1Chamber2 Unit1/9(DC)
  Constant39/1 -> Revised Valve Model Chamber1Chamber2 Unit1/10(Rs)
  Constant40/1 -> Revised Valve Model Chamber1Chamber2 Unit1/11(gma)
  Constant42/1 -> Revised Valve Model Chamber1Chamber2 Unit1/12(Tw)
  Constant1/1 -> Revised Valve Model Chamber1Chamber2 Unit1/13(hC)
  Constant41/1 -> Revised Valve Model Chamber1Chamber2 Unit1/8(AC)
  [TimeStep] -> Revised Valve Model Chamber1Chamber2 Unit1/2(TimeStep)
  [PC2] -> Revised Valve Model Chamber1Chamber2 Unit1/14(PC2)
  [TC2] -> Revised Valve Model Chamber1Chamber2 Unit1/15(TC2)
  Constant67/1 -> Revised Valve Model Chamber1Chamber2 Unit1/16(A)
  Revised Valve Model Chamber1Chamber2 Unit1/2(mdotMax) -> mdot Max Chamber1Chamber2 Unit1/1, Unit Delay3/1
  Add3/1 -> Pressure Difference Tank Unit1/1
  [PC2] -> Add7/1
  [PC1] -> Add7/2
  Add7/1 -> Pressure Difference Chamb. 1 Unit1/1
  [PC1] -> Add9/1
  Add9/1 -> Pressure Difference Inlet Unit1/1
  Revised Valve Model/2(mdotMax) -> Unit Delay2/1, mdot Max Cylinder Unit1/1
  Coulomb & Viscous Friction Unit2/1 -> Gain2/1
  Saturation1/1 -> Add12/1, PTO Friction Unit2/1  "Motion Friction"
  Endstop Forces Unit2/2(F_stop_lo) -> joint F stop low Unit2/1, Add12/2  "Fstop_low"
  cylinder total Length1/1 -> Endstop Forces Unit2/2(Total length)
  Sum9/1 -> Endstop Forces Unit2/1(x(t)), joint position2/1  "Piston Position"
  Endstop Forces Unit2/1(F_stop_hi) -> joint F stop high Unit2/1, Add12/3  "Fstop_high"
  Gain2/1 -> Saturation1/1
  Constant93/1 -> Sum9/1
  Add14/1 -> Sum9/2, Volume Chamber1 Box Unit2/1(x), Revised Valve Model Chamber1Chamber2 Unit2/4(x), Pressure Chamber2 Box Unit2/4(x), [xU2], Volume Chamber2 Box Unit2/1(x), Pressure Chamber1 Box Unit2/4(x), piston position Unit2/1  "x"
  Selector2/1 -> piston velocity Unit2/1, Endstop Forces Unit2/3(xdot(t)), Pressure Chamber1 Box Unit2/3(xdot), Revised Valve Model Chamber1Chamber2 Unit2/3(xdot), Pressure Chamber2 Box Unit2/3(xdot), [xDotU2], Product5/1, Coulomb & Viscous Friction Unit2/1  "Xdot"
  Pressure Chamber1 Box Unit2/1(Pdot) -> Pdot Chamber1 Unit2/1, Discrete-Time Integrator3/1  "pdot(t)"
  Sum4/1 -> Discrete-Time Integrator7/1, Air Mass change rate Chamber1 Unit2/1  "mdot1-mdot2"
  Discrete-Time Integrator7/1 -> Air Mass Chamber1 Unit2/1, Temperature Chamber1 Box Unit2/4(m), Assertion6/1  "chamber1 air mass"
  Discrete-Time Integrator3/1 -> Pressure Chamber1 Box Unit2/1(P), [PC1U2], Revised Valve Model Chamber1Chamber2 Unit2/5(PC1), Sum5/1, Assertion7/1, Pressure Chamber1 Unit2/1, Temperature Chamber1 Box Unit2/1(P)  "Chamber1 Pressure"
  cylinder equilibrium offset position10/1 -> Pressure Chamber1 Box Unit2/8(L)
  Cyl D4/1 -> Pressure Chamber1 Box Unit2/10(D)
  Constant120/1 -> Discrete-Time Integrator7/2
  Constant98/1 -> Pressure Chamber1 Box Unit2/11(Rs)
  Constant109/1 -> Pressure Chamber1 Box Unit2/12(gma)
  Constant118/1 -> Pressure Chamber1 Box Unit2/9(A)
  Constant119/1 -> Pressure Chamber1 Box Unit2/13(Tw)
  Constant85/1 -> Pressure Chamber1 Box Unit2/14(h)
  Constant15/1 -> Discrete-Time Integrator3/2
  Constant77/1 -> Temperature Chamber1 Box Unit2/2(Rs)
  Revised Valve Model Chamber1Chamber2 Unit2/1(MassFlow) -> mdot Chamber1Chamber2 Unit2/1, Sum7/2, Pressure Chamber1 Box Unit2/7(mdot3), Sum4/2, Pressure Chamber2 Box Unit2/6(mdot1)  "mdot(t)"
  Pressure Chamber2 Box Unit2/1(Pdot) -> Pdot Chamber2 Unit2/1, Discrete-Time Integrator8/1  "pdot(t)"
  Volume Chamber2 Box Unit2/1(V) -> Vol Chamber2 Unit2/1, Assertion11/1, Temperature Chamber2 Box Unit2/3(V)  "Chamber2 volume"
  Sum7/1 -> Discrete-Time Integrator9/1, Air Mass change rate Chamber2 Unit2/1
  Discrete-Time Integrator9/1 -> Temperature Chamber2 Box Unit2/4(m), Air Mass Chamber2 Unit2/1, Assertion9/1  "Chamber2 air mass"
  Constant13/1 -> Discrete-Time Integrator9/2
  Temperature Chamber2 Box Unit2/1(T) -> Temp Chamber2 Unit2/1, Pressure Chamber2 Box Unit2/2(T), [TC2U2], Pressure Tank Box Unit2/2(Tin)  "Chamber2 temperature"
  Constant11/1 -> Pressure Chamber2 Box Unit2/8(L)
  Constant12/1 -> Pressure Chamber2 Box Unit2/10(D)
  Constant45/1 -> Discrete-Time Integrator8/2
  Constant71/1 -> Pressure Chamber2 Box Unit2/14(h)
  Constant74/1 -> Pressure Chamber2 Box Unit2/11(Rs)
  Constant75/1 -> Pressure Chamber2 Box Unit2/12(gma)
  Constant76/1 -> Pressure Chamber2 Box Unit2/9(A)
  Constant73/1 -> Pressure Chamber2 Box Unit2/13(Tw)
  Constant88/1 -> Temperature Chamber2 Box Unit2/2(Rs)
  Temperature Chamber1 Box Unit2/1(T) -> Pressure Chamber2 Box Unit2/5(Tin1), Temp Chamber1 Unit2/1, [TC1U2], Pressure Chamber1 Box Unit2/2(T), Revised Valve Model Chamber1Chamber2 Unit2/6(TC1)  "chamber1 temp"
  Revised Valve Model Piston Outlet Unit2/1(MassFlow) -> Revised Valve Tank Outlet Unit2/12(mDotIn), Pressure Chamber2 Box Unit2/7(mdot3), Sum7/1, Sum8/1, Pressure Tank Box Unit2/3(mdot1), mdot Cylinder Unit2/1  "Outlet cylinder"
  Gain3/1 -> Add12/4, Product5/2, Mech_FTO Unit2/1  "Pressure Potential Force"
  Sum5/1 -> Chamber pressure potential Unit2/1, Gain3/1
  Product5/1 -> Energy1/1, Mech_PTO Unit2/1
  Energy1/1 -> Mech_Energy Unit2/1
  Discrete-Time Integrator8/1 -> Pressure Chamber2 Box Unit2/1(P), [PC2U2], Pressure Chamber2 Unit2/1, Assertion8/1, Temperature Chamber2 Box Unit2/1(P), Sum5/2  "Chamber2 Pressure"
  Volume Chamber1 Box Unit2/1(V) -> Vol Chamber1 Unit2/1, Assertion10/1, Temperature Chamber1 Box Unit2/3(V)  "Chamber1 Volume"
  cylinder equilibrium offset position7/1 -> Volume Chamber1 Box Unit2/3(L)
  Constant94/1 -> Volume Chamber1 Box Unit2/2(A)
  cylinder equilibrium offset position8/1 -> Volume Chamber2 Box Unit2/3(L)
  Constant97/1 -> Volume Chamber2 Box Unit2/2(A)
  Pressure Tank Box Unit2/1(Pdot) -> Pdot Tank Unit2/1, Discrete-Time Integrator5/1
  Sum8/1 -> Tank Air Mass change rate Unit2/1, Discrete-Time Integrator6/1  "mdot1-mdot2"
  Discrete-Time Integrator6/1 -> Product3/2, Temperature Tank Box Unit2/4(m), Tank Air Mass Unit2/1  "Tank air mas"
  Constant72/1 -> Discrete-Time Integrator6/2
  Constant78/1 -> Pressure Tank Box Unit2/5(Rs)
  Constant79/1 -> Pressure Tank Box Unit2/6(gma)
  Constant80/1 -> Pressure Tank Box Unit2/7(h)
  Constant81/1 -> Discrete-Time Integrator5/2
  Constant82/1 -> Pressure Tank Box Unit2/8(a)
  Constant86/1 -> Pressure Tank Box Unit2/10(Tw)
  Constant99/1 -> Pressure Tank Box Unit2/9(V)
  Constant83/1 -> Temperature Tank Box Unit2/2(Rs)
  Constant96/1 -> Temperature Tank Box Unit2/3(V)
  Temperature Tank Box Unit2/1(T) -> Temp Tank Unit2/1, Pipe Unit1 to Unit1/2(Tin), Determining Useful Energy1/1(T), Revised Valve Tank Outlet Unit2/4(TT), Pressure Tank Box Unit2/1(T), [TTU2]  "Unit1 Tank temp"
  Discrete-Time Integrator5/1 -> [PTU2], Temperature Tank Box Unit2/1(P), Pressure Tank Unit2/1, Determining Useful Energy1/2(P), Add10/2, Revised Valve Tank Outlet Unit2/3(PT)  "Tank pressure"
  [PP_U2] -> Add10/1, Revised Valve Tank Outlet Unit2/17(PP)
  Constant10/1 -> Revised Valve Model Piston Outlet Unit2/13(hC)
  Constant101/1 -> Revised Valve Model Piston Outlet Unit2/12(Tw)
  Constant95/1 -> Revised Valve Model Piston Outlet Unit2/11(gma)
  Constant92/1 -> Revised Valve Model Piston Outlet Unit2/10(Rs)
  Cyl D5/1 -> Revised Valve Model Piston Outlet Unit2/9(DC)
  Constant100/1 -> Revised Valve Model Piston Outlet Unit2/8(AC)
  cylinder equilibrium offset position12/1 -> Revised Valve Model Piston Outlet Unit2/7(LC)
  [TimeStep] -> Revised Valve Model Piston Outlet Unit2/2(TimeStep)
  Constant102/1 -> Revised Valve Model Piston Outlet Unit2/14(hT)
  Constant103/1 -> Revised Valve Model Piston Outlet Unit2/15(aT)
  Constant104/1 -> Revised Valve Model Piston Outlet Unit2/16(VT)
  [PC2U2] -> Revised Valve Model Piston Outlet Unit2/3(PC)
  [TC2U2] -> Revised Valve Model Piston Outlet Unit2/4(TC)
  [xDotU2] -> Revised Valve Model Piston Outlet Unit2/5(xdot)
  [xU2] -> Revised Valve Model Piston Outlet Unit2/6(x)
  [TTU2] -> Revised Valve Model Piston Outlet Unit2/18(TT)
  [PTU2] -> Add6/1
  [PC2U2] -> Add6/2
  Add6/1 -> Pressure Difference Cyl. Unit2/1
  [PTU2] -> Revised Valve Model Piston Outlet Unit2/17(PT)
  [TimeStep] -> Revised Valve Tank Outlet Unit2/2(TimeStep)
  Constant106/1 -> Revised Valve Tank Outlet Unit2/7(Tw)
  Constant70/1 -> Revised Valve Tank Outlet Unit2/6(gma)
  Constant69/1 -> Revised Valve Tank Outlet Unit2/5(Rs)
  Constant107/1 -> Revised Valve Tank Outlet Unit2/8(hT)
  Constant108/1 -> Revised Valve Tank Outlet Unit2/10(aT)
  Constant110/1 -> Revised Valve Tank Outlet Unit2/9(VT)
  Revised Valve Tank Outlet Unit2/1(MassFlow) -> " mdot Tank Unit2"/1, Sum15/1, Pipe Unit1 to Unit1/3(mdot1), Determining Useful Energy1/3(mDot), Revised Valve Pipe Outlet Unit2/12(mDotIn), Sum8/2, Pressure Tank Box Unit2/4(mdot2)  "Unit1 Outlet tank mdot"
  Constant68/1 -> Revised Valve Tank Outlet Unit2/13(A)
  Revised Valve Tank Outlet Unit2/2(mdotMax) -> Unit Delay5/1, " mdot max Tank Unit2"/1
  Constant116/1 -> Revised Valve Model Piston Outlet Unit2/19(A)
  cylinder equilibrium offset position9/1 -> Revised Valve Model Chamber1Chamber2 Unit2/7(LC)
  Cyl D7/1 -> Revised Valve Model Chamber1Chamber2 Unit2/9(DC)
  Constant87/1 -> Revised Valve Model Chamber1Chamber2 Unit2/10(Rs)
  Constant89/1 -> Revised Valve Model Chamber1Chamber2 Unit2/11(gma)
  Constant91/1 -> Revised Valve Model Chamber1Chamber2 Unit2/12(Tw)
  Constant2/1 -> Revised Valve Model Chamber1Chamber2 Unit2/13(hC)
  Constant90/1 -> Revised Valve Model Chamber1Chamber2 Unit2/8(AC)
  [TimeStep] -> Revised Valve Model Chamber1Chamber2 Unit2/2(TimeStep)
  [PC2U2] -> Revised Valve Model Chamber1Chamber2 Unit2/14(PC2)
  [TC2U2] -> Revised Valve Model Chamber1Chamber2 Unit2/15(TC2)
  Constant117/1 -> Revised Valve Model Chamber1Chamber2 Unit2/16(A)
  Revised Valve Model Chamber1Chamber2 Unit2/2(mdotMax) -> Unit Delay7/1, mdot Max Chamber1Chamber2 Unit2/1
  Add10/1 -> Pressure Difference Tank Unit2/1
  [PC2U2] -> Add11/1
  [PC1U2] -> Add11/2
  Add11/1 -> Pressure Difference Chamb. 1 Unit2/1
  Revised Valve Model Piston Outlet Unit2/2(mdotMax) -> Unit Delay6/1, mdot Max Cylinder Unit2/1
  Coulomb & Viscous Friction Unit3/1 -> Gain4/1
  Saturation2/1 -> PTO Friction Unit3/1, Add19/1  "Motion Friction"
  Endstop Forces Unit3/2(F_stop_lo) -> joint F stop low Unit3/1, Add19/2  "Fstop_low"
  cylinder total Length2/1 -> Endstop Forces Unit3/2(Total length)
  Sum14/1 -> Endstop Forces Unit3/1(x(t)), joint position3/1  "Piston Position"
  Endstop Forces Unit3/1(F_stop_hi) -> joint F stop high Unit3/1, Add19/3  "Fstop_high"
  Gain4/1 -> Saturation2/1
  Constant153/1 -> Sum14/1
  Add15/1 -> Volume Chamber1 Box Unit3/1(x), Revised Valve Model Chamber1Chamber2 Unit3/4(x), Pressure Chamber2 Box Unit3/4(x), [xU3], Volume Chamber2 Box Unit3/1(x), Pressure Chamber1 Box Unit3/4(x), Sum14/2, piston position Unit3/1  "x"
  Selector4/1 -> piston velocity Unit3/1, Coulomb & Viscous Friction Unit3/1, Pressure Chamber1 Box Unit3/3(xdot), Revised Valve Model Chamber1Chamber2 Unit3/3(xdot), Pressure Chamber2 Box Unit3/3(xdot), [xDotU3], Product8/1, Endstop Forces Unit3/3(xdot(t))  "Xdot"
  Pressure Chamber1 Box Unit3/1(Pdot) -> Pdot Chamber1 Unit3/1, Discrete-Time Integrator14/1  "pdot(t)"
  Sum10/1 -> Discrete-Time Integrator17/1, Air Mass change rate Chamber1 Unit3/1  "mdot1-mdot2"
  Discrete-Time Integrator17/1 -> Air Mass Chamber1 Unit3/1, Temperature Chamber1 Box Unit3/4(m), Assertion12/1  "chamber1 air mass"
  Discrete-Time Integrator14/1 -> Pressure Chamber1 Box Unit3/1(P), [PC1U3], Revised Valve Model Chamber1Chamber2 Unit3/5(PC1), Sum11/1, Assertion13/1, Pressure Chamber1 Unit3/1, Temperature Chamber1 Box Unit3/1(P)  "Chamber1 Pressure"
  cylinder equilibrium offset position16/1 -> Pressure Chamber1 Box Unit3/8(L)
  Cyl D8/1 -> Pressure Chamber1 Box Unit3/10(D)
  Constant180/1 -> Discrete-Time Integrator17/2
  Constant158/1 -> Pressure Chamber1 Box Unit3/11(Rs)
  Constant169/1 -> Pressure Chamber1 Box Unit3/12(gma)
  Constant178/1 -> Pressure Chamber1 Box Unit3/9(A)
  Constant179/1 -> Pressure Chamber1 Box Unit3/13(Tw)
  Constant145/1 -> Pressure Chamber1 Box Unit3/14(h)
  Constant126/1 -> Discrete-Time Integrator14/2
  Constant137/1 -> Temperature Chamber1 Box Unit3/2(Rs)
  Revised Valve Model Chamber1Chamber2 Unit3/1(MassFlow) -> mdot Chamber1Chamber2 Unit3/1, Sum12/2, Pressure Chamber1 Box Unit3/7(mdot3), Sum10/2, Pressure Chamber2 Box Unit3/6(mdot1)  "mdot(t)"
  Pressure Chamber2 Box Unit3/1(Pdot) -> Pdot Chamber2 Unit3/1, Discrete-Time Integrator18/1  "pdot(t)"
  Volume Chamber2 Box Unit3/1(V) -> Vol Chamber2 Unit3/1, Assertion17/1, Temperature Chamber2 Box Unit3/3(V)  "Chamber2 volume"
  Sum12/1 -> Discrete-Time Integrator19/1, Air Mass change rate Chamber2 Unit3/1
  Discrete-Time Integrator19/1 -> Temperature Chamber2 Box Unit3/4(m), Air Mass Chamber2 Unit3/1, Assertion15/1  "Chamber2 air mass"
  Constant125/1 -> Discrete-Time Integrator19/2
  Temperature Chamber2 Box Unit3/1(T) -> Temp Chamber2 Unit3/1, Pressure Chamber2 Box Unit3/2(T), [TC2U3], Pressure Tank Box Unit3/2(Tin)  "Chamber2 temperature"
  Constant123/1 -> Pressure Chamber2 Box Unit3/8(L)
  Constant124/1 -> Pressure Chamber2 Box Unit3/10(D)
  Constant127/1 -> Discrete-Time Integrator18/2
  Constant131/1 -> Pressure Chamber2 Box Unit3/14(h)
  Constant134/1 -> Pressure Chamber2 Box Unit3/11(Rs)
  Constant135/1 -> Pressure Chamber2 Box Unit3/12(gma)
  Constant136/1 -> Pressure Chamber2 Box Unit3/9(A)
  Constant133/1 -> Pressure Chamber2 Box Unit3/13(Tw)
  Constant148/1 -> Temperature Chamber2 Box Unit3/2(Rs)
  Temperature Chamber1 Box Unit3/1(T) -> Pressure Chamber2 Box Unit3/5(Tin1), Temp Chamber1 Unit3/1, [TC1U3], Pressure Chamber1 Box Unit3/2(T), Revised Valve Model Chamber1Chamber2 Unit3/6(TC1)  "chamber1 temp"
  Revised Valve Model Piston Outlet Unit3/1(MassFlow) -> Revised Valve Tank Outlet2/13(mDotIn), Pressure Chamber2 Box Unit3/7(mdot3), Sum12/1, Sum13/1, Pressure Tank Box Unit3/3(mdot1), mdot Cylinder Unit3/1  "Outlet cylinder"
  Gain5/1 -> Add19/4, Product8/2, Mech_FTO Unit3/1  "Pressure Potential Force"
  Sum11/1 -> Chamber pressure potential Unit3/1, Gain5/1
  Product8/1 -> Energy2/1, Mech_PTO Unit3/1
  Energy2/1 -> Mech_Energy Unit3/1
  Discrete-Time Integrator18/1 -> Pressure Chamber2 Box Unit3/1(P), [PC2U3], Pressure Chamber2 Unit3/1, Assertion14/1, Temperature Chamber2 Box Unit3/1(P), Sum11/2  "Chamber2 Pressure"
  Volume Chamber1 Box Unit3/1(V) -> Vol Chamber1 Unit3/1, Assertion16/1, Temperature Chamber1 Box Unit3/3(V)  "Chamber1 Volume"
  cylinder equilibrium offset position13/1 -> Volume Chamber1 Box Unit3/3(L)
  Constant154/1 -> Volume Chamber1 Box Unit3/2(A)
  cylinder equilibrium offset position14/1 -> Volume Chamber2 Box Unit3/3(L)
  Constant157/1 -> Volume Chamber2 Box Unit3/2(A)
  Pressure Tank Box Unit3/1(Pdot) -> Pdot Tank Unit3/1, Discrete-Time Integrator15/1
  Sum13/1 -> Tank Air Mass change rate Unit3/1, Discrete-Time Integrator16/1  "mdot1-mdot2"
  Discrete-Time Integrator16/1 -> Temperature Tank Box Unit3/4(m), Product4/2, Tank Air Mass Unit3/1  "Tank air mas"
  Constant132/1 -> Discrete-Time Integrator16/2
  Constant138/1 -> Pressure Tank Box Unit3/5(Rs)
  Constant139/1 -> Pressure Tank Box Unit3/6(gma)
  Constant140/1 -> Pressure Tank Box Unit3/7(h)
  Constant141/1 -> Discrete-Time Integrator15/2
  Constant142/1 -> Pressure Tank Box Unit3/8(a)
  Constant146/1 -> Pressure Tank Box Unit3/10(Tw)
  Constant159/1 -> Pressure Tank Box Unit3/9(V)
  Constant143/1 -> Temperature Tank Box Unit3/2(Rs)
  Constant156/1 -> Temperature Tank Box Unit3/3(V)
  Temperature Tank Box Unit3/1(T) -> Temp Tank Unit3/1, Determining Useful Energy2/1(T), Revised Valve Tank Outlet2/4(TT), Pressure Tank Box Unit3/1(T), [TTU3]  "Unit1 Tank temp"
  Discrete-Time Integrator15/1 -> [PTU3], Temperature Tank Box Unit3/1(P), Pressure Tank Unit3/1, Revised Valve Tank Outlet2/3(PT), Determining Useful Energy2/2(P), Add17/2  "Tank pressure"
  override3/1 -> Add17/1, Revised Valve Tank Outlet2/11(Pcrack)
  Constant122/1 -> Revised Valve Model Piston Outlet Unit3/13(hC)
  Constant161/1 -> Revised Valve Model Piston Outlet Unit3/12(Tw)
  Constant155/1 -> Revised Valve Model Piston Outlet Unit3/11(gma)
  Constant152/1 -> Revised Valve Model Piston Outlet Unit3/10(Rs)
  Cyl D9/1 -> Revised Valve Model Piston Outlet Unit3/9(DC)
  Constant160/1 -> Revised Valve Model Piston Outlet Unit3/8(AC)
  cylinder equilibrium offset position18/1 -> Revised Valve Model Piston Outlet Unit3/7(LC)
  [TimeStep] -> Revised Valve Model Piston Outlet Unit3/2(TimeStep)
  Constant162/1 -> Revised Valve Model Piston Outlet Unit3/14(hT)
  Constant163/1 -> Revised Valve Model Piston Outlet Unit3/15(aT)
  Constant164/1 -> Revised Valve Model Piston Outlet Unit3/16(VT)
  [PC2U3] -> Revised Valve Model Piston Outlet Unit3/3(PC)
  [TC2U3] -> Revised Valve Model Piston Outlet Unit3/4(TC)
  [xDotU3] -> Revised Valve Model Piston Outlet Unit3/5(xdot)
  [xU3] -> Revised Valve Model Piston Outlet Unit3/6(x)
  [TTU3] -> Revised Valve Model Piston Outlet Unit3/18(TT)
  [PTU3] -> Add16/1
  [PC2U3] -> Add16/2
  Add16/1 -> Pressure Difference Cyl. Unit3/1
  [PTU3] -> Revised Valve Model Piston Outlet Unit3/17(PT)
  [TimeStep] -> Revised Valve Tank Outlet2/2(TimeStep)
  Constant166/1 -> Revised Valve Tank Outlet2/7(Tw)
  Constant130/1 -> Revised Valve Tank Outlet2/6(gma)
  Constant129/1 -> Revised Valve Tank Outlet2/5(Rs)
  Constant167/1 -> Revised Valve Tank Outlet2/8(hT)
  Constant168/1 -> Revised Valve Tank Outlet2/10(aT)
  Constant170/1 -> Revised Valve Tank Outlet2/9(VT)
  [TC2U3] -> Revised Valve Tank Outlet2/12(TC)
  Revised Valve Tank Outlet2/1(MassFlow) -> " mdot Tank Unit3"/1, Determining Useful Energy2/3(mDot), Sum13/2, Pressure Tank Box Unit3/4(mdot2)  "Unit1 Outlet tank mdot"
  Constant128/1 -> Revised Valve Tank Outlet2/14(A)
  Revised Valve Tank Outlet2/2(mdotMax) -> Unit Delay8/1, " mdot max Tank Unit3"/1
  Constant176/1 -> Revised Valve Model Piston Outlet Unit3/19(A)
  cylinder equilibrium offset position15/1 -> Revised Valve Model Chamber1Chamber2 Unit3/7(LC)
  Cyl D11/1 -> Revised Valve Model Chamber1Chamber2 Unit3/9(DC)
  Constant147/1 -> Revised Valve Model Chamber1Chamber2 Unit3/10(Rs)
  Constant149/1 -> Revised Valve Model Chamber1Chamber2 Unit3/11(gma)
  Constant151/1 -> Revised Valve Model Chamber1Chamber2 Unit3/12(Tw)
  Constant121/1 -> Revised Valve Model Chamber1Chamber2 Unit3/13(hC)
  Constant150/1 -> Revised Valve Model Chamber1Chamber2 Unit3/8(AC)
  [TimeStep] -> Revised Valve Model Chamber1Chamber2 Unit3/2(TimeStep)
  [PC2U3] -> Revised Valve Model Chamber1Chamber2 Unit3/14(PC2)
  [TC2U3] -> Revised Valve Model Chamber1Chamber2 Unit3/15(TC2)
  Constant177/1 -> Revised Valve Model Chamber1Chamber2 Unit3/16(A)
  Revised Valve Model Chamber1Chamber2 Unit3/2(mdotMax) -> Unit Delay10/1, mdot Max Chamber1Chamber2 Unit3/1
  Add17/1 -> Pressure Difference Tank Unit3/1
  [PC2U3] -> Add18/1
  [PC1U3] -> Add18/2
  Add18/1 -> Pressure Difference Chamb. 1 Unit3/1
  Revised Valve Model Piston Outlet Unit3/2(mdotMax) -> Unit Delay9/1, mdot Max Cylinder Unit3/1
  Constant111/1 -> Revised Valve Tank Outlet Unit1/16(hP)
  [PP] -> Revised Valve Tank Outlet Unit1/17(PP), Add3/1
  Unit Delay/1 -> Revised Valve Tank Outlet Unit1/1(mdotMaxOld)
  Unit Delay2/1 -> Revised Valve Model/1(mdotMaxOld)
  Unit Delay3/1 -> Revised Valve Model Chamber1Chamber2 Unit1/1(mdotMaxOld)
  Unit Delay4/1 -> Revised Valve Model Inlet Unit1/1(mdotMaxOld)
  Unit Delay5/1 -> Revised Valve Tank Outlet Unit2/1(mdotMaxOld)
  Unit Delay6/1 -> Revised Valve Model Piston Outlet Unit2/1(mdotMaxOld)
  Unit Delay7/1 -> Revised Valve Model Chamber1Chamber2 Unit2/1(mdotMaxOld)
  Unit Delay8/1 -> Revised Valve Tank Outlet2/1(mdotMaxOld)
  Unit Delay9/1 -> Revised Valve Model Piston Outlet Unit3/1(mdotMaxOld)
  Unit Delay10/1 -> Revised Valve Model Chamber1Chamber2 Unit3/1(mdotMaxOld)
  Product1/1 -> Determining Useful Energy/4(Density)
  Constant114/1 -> Determining Useful Energy/6(Rs)
  Atmospheric pressure2/1 -> Determining Useful Energy/8(Pamb)
  tempAmb2/1 -> Determining Useful Energy/7(Tamb)
  Constant115/1 -> Determining Useful Energy/5(Cp)
  Determining Useful Energy/1(Exergy) -> Exergy Unit1/1
  Determining Useful Energy/2(Power) -> Energy Unit1/1
  Constant36/1 -> Product1/1
  Product3/1 -> Determining Useful Energy1/4(Density)
  Constant165/1 -> Determining Useful Energy1/6(Rs)
  Atmospheric pressure3/1 -> Determining Useful Energy1/8(Pamb)
  tempAmb3/1 -> Determining Useful Energy1/7(Tamb)
  Constant171/1 -> Determining Useful Energy1/5(Cp)
  Determining Useful Energy1/1(Exergy) -> Exergy Unit2/1
  Determining Useful Energy1/2(Power) -> Energy Unit2/1
  Constant84/1 -> Product3/1
  Constant172/1 -> Determining Useful Energy2/6(Rs)
  Atmospheric pressure4/1 -> Determining Useful Energy2/8(Pamb)
  tempAmb4/1 -> Determining Useful Energy2/7(Tamb)
  Constant173/1 -> Determining Useful Energy2/5(Cp)
  Determining Useful Energy2/1(Exergy) -> Exergy Unit3/1
  Determining Useful Energy2/2(Power) -> Energy Unit3/1
  Constant144/1 -> Product4/1
  Product4/1 -> Determining Useful Energy2/4(Density)
  Pipe Unit1 to Unit2/1(Pdot) -> Pdot Pipe U1U2/1, Discrete-Time Integrator21/1
  Sum16/1 -> Pipe Air Mass change rate U1U2/1, Discrete-Time Integrator20/1  "mdot1-mdot2"
  Discrete-Time Integrator20/1 -> Temperature Pipe Unit1 to Unit2/4(m), Air Mass Pipe U1U2/1  "Tank air mas"
  Constant201/1 -> Discrete-Time Integrator20/2
  Constant202/1 -> Pipe Unit1 to Unit2/5(Rs)
  Constant203/1 -> Pipe Unit1 to Unit2/6(gma)
  Constant204/1 -> Pipe Unit1 to Unit2/7(h)
  Constant205/1 -> Discrete-Time Integrator21/2
  Constant206/1 -> Pipe Unit1 to Unit2/8(a)
  Constant209/1 -> Pipe Unit1 to Unit2/10(Tw)
  Constant220/1 -> Pipe Unit1 to Unit2/9(V)
  Constant207/1 -> Temperature Pipe Unit1 to Unit2/2(Rs)
  Constant212/1 -> Temperature Pipe Unit1 to Unit2/3(V)
  Temperature Pipe Unit1 to Unit2/1(T) -> Temp Pipe U1U2/1, Pipe Unit1 to Unit2/1(T), [TP], Pressure Chamber1 Box Unit2/5(Tin1), Revised Valve Pipe Outlet Unit1/4(TP)  "Unit1 Tank temp"
  Discrete-Time Integrator21/1 -> [PP], Add5/2, Revised Valve Pipe Outlet Unit1/3(PP), Temperature Pipe Unit1 to Unit2/1(P), Pressure Pipe U1U2/1  "Tank pressure"
  [TimeStep] -> Revised Valve Pipe Outlet Unit1/2(TimeStep)
  Constant214/1 -> Revised Valve Pipe Outlet Unit1/7(Tw)
  Constant213/1 -> Revised Valve Pipe Outlet Unit1/6(gma)
  Constant211/1 -> Revised Valve Pipe Outlet Unit1/5(Rs)
  Constant215/1 -> Revised Valve Pipe Outlet Unit1/8(hP)
  Constant216/1 -> Revised Valve Pipe Outlet Unit1/10(aP)
  Constant217/1 -> Revised Valve Pipe Outlet Unit1/9(VP)
  [TT] -> Revised Valve Pipe Outlet Unit1/11(TT)
  Revised Valve Pipe Outlet Unit1/1(MassFlow) -> " mdot Pipe U1U2"/1, Sum4/1, Pressure Chamber1 Box Unit2/6(mdot1), Sum16/2, Pipe Unit1 to Unit2/4(mdot2)  "Unit1 Outlet pipe mdot"
  Constant210/1 -> Revised Valve Pipe Outlet Unit1/13(A)
  Revised Valve Pipe Outlet Unit1/2(mdotMax) -> Unit Delay12/1, " mdot max Pipe U1U2"/1
  Add5/1 -> Pressure Difference Pipe Unit1/1
  cylinder equilibrium offset position20/1 -> Revised Valve Pipe Outlet Unit1/17(LC)
  Constant200/1 -> Revised Valve Pipe Outlet Unit1/14(AC)
  Cyl D13/1 -> Revised Valve Pipe Outlet Unit1/19(DC)
  Constant208/1 -> Revised Valve Pipe Outlet Unit1/18(hC)
  [xU2] -> Revised Valve Pipe Outlet Unit1/15(x)
  [xDotU2] -> Revised Valve Pipe Outlet Unit1/16(xDot)
  [PC1U2] -> Add5/1, Revised Valve Pipe Outlet Unit1/20(PC1)
  [TC1U2] -> Revised Valve Pipe Outlet Unit1/21(TC1)
  Unit Delay12/1 -> Revised Valve Pipe Outlet Unit1/1(mdotMaxOld)
  [TP] -> Revised Valve Tank Outlet Unit1/18(TP)
  Constant105/1 -> Revised Valve Tank Outlet Unit1/15(aP)
  Constant218/1 -> Revised Valve Tank Outlet Unit1/14(VP)
  [PC1U3] -> Revised Valve Pipe Outlet Unit2/20(PC1), Add4/1
  [TimeStep] -> Revised Valve Pipe Outlet Unit2/2(TimeStep)
  Revised Valve Pipe Outlet Unit2/1(MassFlow) -> " mdot Pipe U2U3"/1, Sum10/1, Pressure Chamber1 Box Unit3/6(mdot1), Sum15/2, Pipe Unit1 to Unit1/4(mdot2)  "Unit1 Outlet pipe mdot"
  Constant196/1 -> Revised Valve Pipe Outlet Unit2/13(A)
  Revised Valve Pipe Outlet Unit2/2(mdotMax) -> Unit Delay11/1, " mdot max Pipe U2U3"/1
  Add4/1 -> Pressure Difference Pipe U2U3/1
  cylinder equilibrium offset position11/1 -> Revised Valve Pipe Outlet Unit2/17(LC)
  Constant194/1 -> Revised Valve Pipe Outlet Unit2/14(AC)
  Cyl D6/1 -> Revised Valve Pipe Outlet Unit2/19(DC)
  [xU3] -> Revised Valve Pipe Outlet Unit2/15(x)
  [TC1U3] -> Revised Valve Pipe Outlet Unit2/21(TC1)
  Constant195/1 -> Revised Valve Pipe Outlet Unit2/18(hC)
  [xDotU3] -> Revised Valve Pipe Outlet Unit2/16(xDot)
  Unit Delay11/1 -> Revised Valve Pipe Outlet Unit2/1(mdotMaxOld)
  Pipe Unit1 to Unit1/1(Pdot) -> Pdot Pipe U2U3/1, Discrete-Time Integrator13/1
  Sum15/1 -> Pipe Air Mass change rate U2U3/1, Discrete-Time Integrator4/1  "mdot1-mdot2"
  Discrete-Time Integrator4/1 -> Temperature Pipe Unit1 to Unit1/4(m), Air Mass Pipe U2U3/1  "Tank air mas"
  Constant112/1 -> Discrete-Time Integrator4/2
  Constant175/1 -> Pipe Unit1 to Unit1/5(Rs)
  Constant181/1 -> Pipe Unit1 to Unit1/6(gma)
  Constant182/1 -> Pipe Unit1 to Unit1/7(h)
  Constant183/1 -> Discrete-Time Integrator13/2
  Constant184/1 -> Pipe Unit1 to Unit1/8(a)
  Constant186/1 -> Pipe Unit1 to Unit1/10(Tw)
  Constant188/1 -> Pipe Unit1 to Unit1/9(V)
  Constant185/1 -> Temperature Pipe Unit1 to Unit1/2(Rs)
  Constant187/1 -> Temperature Pipe Unit1 to Unit1/3(V)
  Temperature Pipe Unit1 to Unit1/1(T) -> Temp Pipe U2U3/1, Pipe Unit1 to Unit1/1(T), [TP_U2], Pressure Chamber1 Box Unit3/5(Tin1), Revised Valve Pipe Outlet Unit2/4(TP)  "Unit1 Tank temp"
  Discrete-Time Integrator13/1 -> Add4/2, Revised Valve Pipe Outlet Unit2/3(PP), [PP_U2], Temperature Pipe Unit1 to Unit1/1(P), Pressure Pipe U2U3/1  "Tank pressure"
  Constant197/1 -> Revised Valve Pipe Outlet Unit2/5(Rs)
  Constant198/1 -> Revised Valve Pipe Outlet Unit2/6(gma)
  Constant174/1 -> Revised Valve Pipe Outlet Unit2/7(Tw)
  Constant189/1 -> Revised Valve Pipe Outlet Unit2/8(hP)
  Constant193/1 -> Revised Valve Pipe Outlet Unit2/9(VP)
  Constant190/1 -> Revised Valve Pipe Outlet Unit2/10(aP)
  [TTU2] -> Revised Valve Pipe Outlet Unit2/11(TT)
  [TC2U2] -> Revised Valve Tank Outlet Unit2/11(TC)
  [TP_U2] -> Revised Valve Tank Outlet Unit2/18(TP)
  Constant191/1 -> Revised Valve Tank Outlet Unit2/16(hP)
  Constant113/1 -> Revised Valve Tank Outlet Unit2/15(aP)
  Constant199/1 -> Revised Valve Tank Outlet Unit2/14(VP)
  cylinder total Length3/1 -> Add13/2
  cylinder total Length4/1 -> Add14/2
  Selector3/1 -> Add14/1  "x"
  cylinder total Length5/1 -> Add15/2
  Selector5/1 -> Add15/1
  Add8/1 -> Gain8/1, Total Reaction Force/1  "Total Reaction Force"
  Bus Selector/1 -> Gain7/1  "<velocity>"
  Gain8/1 -> Translational PTO Actuation Force/1
  Gain6/1 -> Selector1/1
  Selector1/1 -> Add13/1
  Bus Selector/2 -> Gain6/1  "<position>"
  Gain7/1 -> Selector/1
  Translational PTO Actuation Force/1 -> Bus Selector/1
  Selector/1 -> Coulomb & Viscous Friction Unit1/1, Endstop Forces Unit1/3(xdot(t)), Pressure Chamber1 Box Unit1/3(xdot), Revised Valve Model Chamber1Chamber2 Unit1/3(xdot), Product2/1, Pressure Chamber2 Box Unit1/3(xdot), [xDot], piston velocity Unit4/1
  Add12/1 -> Gain11/1, Total Reaction Force1/1  "Total Reaction Force"
  Bus Selector1/1 -> Gain10/1  "<velocity>"
  Gain11/1 -> Translational PTO Actuation Force1/1
  Gain9/1 -> Selector3/1
  Bus Selector1/2 -> Gain9/1  "<position>"
  Gain10/1 -> Selector2/1
  Translational PTO Actuation Force1/1 -> Bus Selector1/1
  Bus Selector2/2 -> Gain14/1  "<position>"
  Gain12/1 -> Selector4/1
  Gain14/1 -> Selector5/1
  Bus Selector2/1 -> Gain12/1  "<velocity>"
  Translational PTO Actuation Force2/1 -> Bus Selector2/1
  Add19/1 -> Total Reaction Force2/1, Gain13/1  "Total Reaction Force"
  Gain13/1 -> Translational PTO Actuation Force2/1
  connections:
  Floating (6DOF)/RConn1 -- Spar/RConn1 -- Translational PTO Actuation Force/LConn1
  Floating (6DOF)/LConn1 -- Floating (6DOF)2/LConn1 -- Floating (6DOF)1/LConn1 -- Global Reference Frame/RConn1
  Translational PTO Actuation Force/RConn1 -- Float/RConn1
  Spar1/RConn1 -- Floating (6DOF)1/RConn1 -- Translational PTO Actuation Force1/LConn1
  Float1/RConn1 -- Translational PTO Actuation Force1/RConn1
  Translational PTO Actuation Force2/LConn1 -- Floating (6DOF)2/RConn1 -- Spar2/RConn1
  Float2/RConn1 -- Translational PTO Actuation Force2/RConn1
